simulink model "fourinputslq_and_yaw_rate_control_sim"  (R2014b)
settings: Solver=ode45  SolverMode=SingleTasking  StartTime=0.0  StopTime=10.0  MaxStep=0.01  RelTol=1e-3
values from neighbouring files (symbols this model uses):
  A = eval(As)    [fourinputslq_and_yaw_rate_control.m]
  B = eval(Bs)    [fourinputslq_and_yaw_rate_control.m]
  Cs = [1 0 0 0 0 0; 0 1 0 0 0 0; 0 0 1 0 0 0;  0 0 0 1 0 0;0 0 0 0 1 0]    [fourinputslq_and_yaw_rate_control.m]
  Kr = -inv(Cc*inv(Aa-Bb*K)*Bb(:,2:4))    [fourinputslq_and_yaw_rate_control.m]
undefined symbols (not defined in the file or in its folder): K
settings Model: CovSFcnEnable=on  Creator=Jaby  LastModifiedBy=danielpihlquist
settings OptimizationCC: BlockReduction=off  BooleanDataType=off  UseDivisionForNetSlopeComputation=off  SimCompilerOptimization=off
settings DebuggingCC: SaveWithParameterizedLinksMsg=none  UnderspecifiedInitializationDetection=Classic  MergeDetectMultiDrivingBlocksExec=none  SignalResolutionControl=TryResolveAllWithWarning  SolverPrmCheckMsg=none  FrameProcessingCompatibilityMsg=error
settings HardwareCC: TargetUnknown=on
settings RTWCC: RTWCompilerOptimization=off

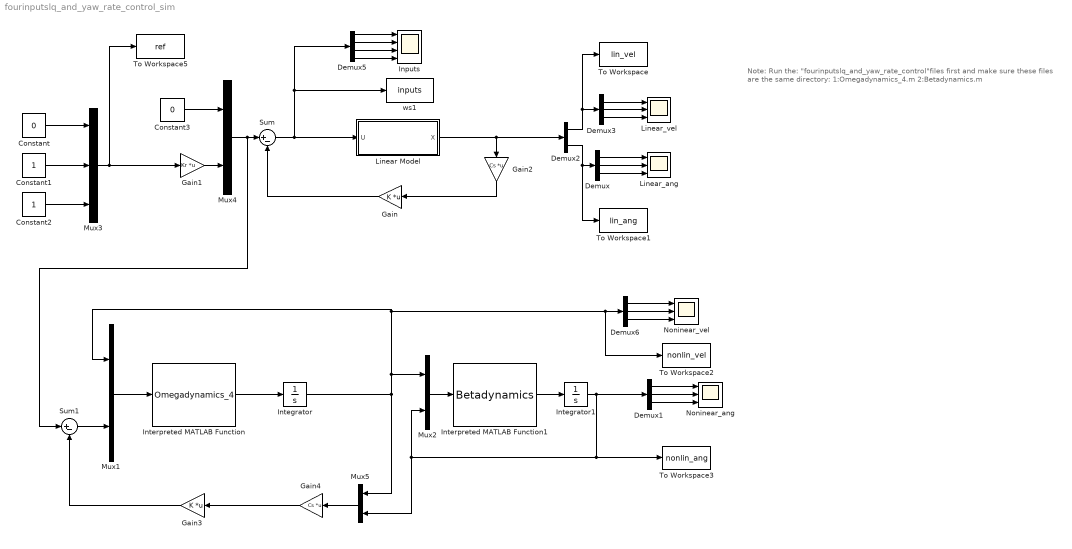
== system fourinputslq_and_yaw_rate_control_sim ==
  note: Note:
      | Run the: "fourinputslq_and_yaw_rate_control"files first and make sure these files are the same directory:
      | 1:Omegadynamics_4.m
      | 2:Betadynamics.m
  Constant : Constant  Value=0
  Constant1 : Constant
  Constant2 : Constant
  Constant3 : Constant  Value=0  VectorParams1D=off
  Demux{,1,3,6} (4 alike) : Demux  Outputs=3
  Demux2 : Demux  Outputs=2
  Demux5 : Demux
  Gain : Gain  Gain=K  Multiplication=Matrix(K*u)
  Gain1 : Gain  Gain=Kr  Multiplication=Matrix(K*u)
  Gain2 : Gain  Gain=Cs  Multiplication=Matrix(K*u)
  Gain3 : Gain  Gain=K  Multiplication=Matrix(K*u)
  Gain4 : Gain  Gain=Cs  Multiplication=Matrix(K*u)
  Inputs : Scope  NumInputPorts=4
      settings: TimeRange=20  YMin=0.00274~-3.07e-14~8.3e-31~-5  YMax=0.00278~-3.025e-14~8.43e-31~5  SaveName=ScopeData4
  Integrator : Integrator  InitialCondition=[0 0 0]'
  Integrator1 : Integrator  InitialCondition=[0 0 0]'
  Interpreted MATLAB Function : MATLABFcn  MATLABFcn=Omegadynamics_4  Output1D=off
  Interpreted MATLAB Function1 : MATLABFcn  MATLABFcn=Betadynamics  Output1D=off
  "Linear Model " : Subsystem
  Linear_ang : Scope  NumInputPorts=3
      settings: TimeRange=20  YMin=0.00274~-3.07e-14~8.3e-31  YMax=0.00278~-3.025e-14~8.43e-31
  Linear_vel : Scope  NumInputPorts=3
      settings: TimeRange=20  YMin=-0.5~-0.5~0  YMax=2.5~2.5~0.7000000000000001  SaveName=ScopeData2
  Mux{1..2,4..5} (4 alike) : Mux  Inputs=2
  Mux3 : Mux  Inputs=3
  Noninear_ang : Scope  NumInputPorts=3
      settings: TimeRange=20  YMin=0.00274~-3.07e-14~8.3e-31  YMax=0.00278~-3.025e-14~8.43e-31
  Noninear_vel : Scope  NumInputPorts=3
      settings: TimeRange=20  YMin=0.00274~-3.07e-14~8.3e-31  YMax=0.00278~-3.025e-14~8.43e-31  SaveName=ScopeData5
  Sum : Sum  Inputs=|+-
  Sum1 : Sum  Inputs=|+-
  To Workspace : ToWorkspace  VariableName=lin_vel  SampleTime=-1
  To Workspace1 : ToWorkspace  VariableName=lin_ang  SampleTime=-1
  To Workspace2 : ToWorkspace  VariableName=nonlin_vel  SampleTime=-1
  To Workspace3 : ToWorkspace  VariableName=nonlin_ang  SampleTime=-1
  To Workspace5 : ToWorkspace  VariableName=ref  SampleTime=-1
  ws1 : ToWorkspace  VariableName=inputs  SampleTime=-1
  wires:
  Demux/1 -> Linear_ang/1
  Demux/2 -> Linear_ang/2
  Demux/3 -> Linear_ang/3
  Integrator/1 -> To Workspace2/1, Demux6/1, Mux1/1, Mux2/1, Mux5/1
  Mux1/1 -> Interpreted MATLAB Function/1
  Interpreted MATLAB Function/1 -> Integrator/1
  Interpreted MATLAB Function1/1 -> Integrator1/1
  Gain/1 -> Sum/2
  Demux2/2 -> To Workspace1/1, Demux/1
  Constant1/1 -> Mux3/2
  Constant/1 -> Mux3/1
  Demux3/1 -> Linear_vel/1
  Demux3/2 -> Linear_vel/2
  Demux3/3 -> Linear_vel/3
  Constant2/1 -> Mux3/3
  "Linear Model "/1(X) -> Demux2/1, Gain2/1
  Mux4/1 -> Sum1/1, Sum/1
  Gain1/1 -> Mux4/2
  Constant3/1 -> Mux4/1
  Demux5/1 -> Inputs/1
  Demux5/2 -> Inputs/2
  Demux5/3 -> Inputs/3
  Sum/1 -> Demux5/1, ws1/1, "Linear Model "/1(U)
  Gain2/1 -> Gain/1
  Gain4/1 -> Gain3/1
  Gain3/1 -> Sum1/2
  Sum1/1 -> Mux1/2
  Mux5/1 -> Gain4/1
  Mux2/1 -> Interpreted MATLAB Function1/1
  Mux3/1 -> Gain1/1, To Workspace5/1
  Demux2/1 -> Demux3/1, To Workspace/1
  Demux1/1 -> Noninear_ang/1
  Demux1/2 -> Noninear_ang/2
  Demux1/3 -> Noninear_ang/3
  Integrator1/1 -> Demux1/1, To Workspace3/1, Mux2/2, Mux5/2
  Demux6/1 -> Noninear_vel/1
  Demux6/2 -> Noninear_vel/2
  Demux6/3 -> Noninear_vel/3
  Demux5/4 -> Inputs/4

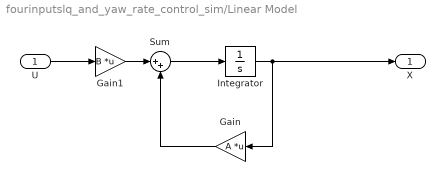
== system fourinputslq_and_yaw_rate_control_sim/Linear Model  ==
  U : Inport
  Gain : Gain  Gain=A  Multiplication=Matrix(K*u)
  Gain1 : Gain  Gain=B  Multiplication=Matrix(K*u)
  Integrator : Integrator
  Sum : Sum  Inputs=|++
  X : Outport
  wires:
  Integrator/1 -> X/1, Gain/1
  U/1 -> Gain1/1
  Gain1/1 -> Sum/1
  Sum/1 -> Integrator/1
  Gain/1 -> Sum/2
